simulink model "simulacao_modelos_discretos"  (R2018b)
settings: Solver=VariableStepAuto  StartTime=0.0  StopTime=15000  FixedStep=5  RelTol=1e-3
values from neighbouring files (symbols this model uses):
  sp_h3 = 0.48    [modelos.mat]    (also in termos_de_Ad.m = sp_h3*1e-2; validacao_tanques.m)
  sp_u = 33.8926009305    [modelos.mat]    (also in termos_de_Ad.m = (sp_q-357.3)/16.4; validacao_tanques.m = (sp_q-357.3)/16.4)
  T = 5.2632    [termos_de_Ad.m]
undefined symbols (not defined in the file or in its folder): Ad, Bd, Cd, Dd
settings Model: Creator=tarsis  LastModifiedBy=tarsis

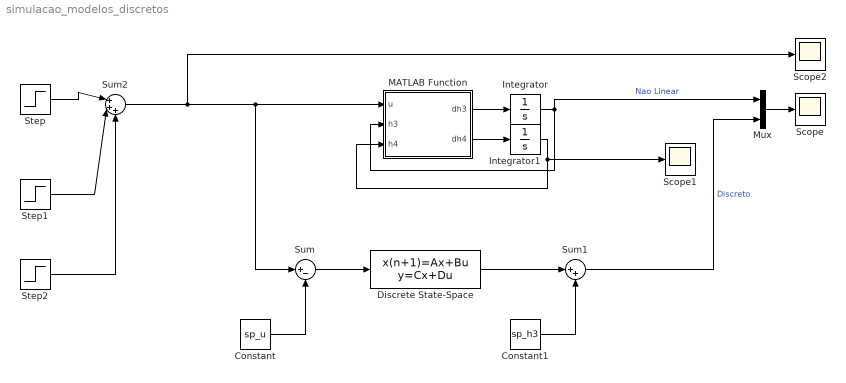
== system simulacao_modelos_discretos ==
  Constant : Constant  Value=sp_u
  Constant1 : Constant  Value=sp_h3
  Discrete State-Space : DiscreteStateSpace  A=Ad  B=Bd  C=Cd  D=Dd  SampleTime=T
  Integrator : Integrator
  Integrator1 : Integrator
  MATLAB Function : MATLAB Function  TreatAsAtomicUnit=on
  Mux : Mux  Inputs=2
  Scope : Scope
  Scope1 : Scope
  Scope2 : Scope
  Step : Step  Time=0  After=sp_u  SampleTime=T
  Step1 : Step  Time=5000  After=-sp_u*0.01  SampleTime=T
  Step2 : Step  Time=10000  After=sp_u*0.02  SampleTime=T
  Sum : Sum  Inputs=|+-
  Sum1 : Sum  Inputs=|++
  Sum2 : Sum  Inputs=|+++
  wires:
  MATLAB Function/1(dh3) -> Integrator/1
  MATLAB Function/2(dh4) -> Integrator1/1
  Integrator/1 -> Mux/1, MATLAB Function/2(h3)  "Nao Linear"
  Integrator1/1 -> Scope1/1, MATLAB Function/3(h4)
  Sum/1 -> Discrete State-Space/1
  Discrete State-Space/1 -> Sum1/1
  Constant/1 -> Sum/2
  Constant1/1 -> Sum1/2
  Mux/1 -> Scope/1
  Sum1/1 -> Mux/2  "Discreto"
  Step/1 -> Sum2/1
  Sum2/1 -> Scope2/1, Sum/1, MATLAB Function/1(u)
  Step1/1 -> Sum2/2
  Step2/1 -> Sum2/3

== matlab function simulacao_modelos_discretos/MATLAB Function ==
  data: u input; dh3 output; dh4 output; h3 input; h4 input
function [dh3,dh4] = fcn(u,h3,h4)
qi = (16.4*u + 357.3)*1e-6;
q12 = 33.51e-4*(h4 - h3) + 43.12e-5;
qout = (87.07e-5*sqrt(h3) + 30.99e-5);
A1 = (pi*(31)^2)*1e-4;
A2 = - 0.88629272879272778105782609278436*h3^16 + 6.0267905557905489111932174309337*h3^15 - 20.80464391736738395516887057851*h3^14 + 47.68494439008527766774004035511*h3^13 - 82.573907447205791291786792565001*h3^12 + 116.28257881925208875326233578017*h3^11 - 139.30893428077013388311346843447*h3^10 + 144.80767028205944702410747888441*h3^9 - 129.2475129476872169884635810807*h3^8 + 96.099152680911332924853135955618*h3^7 - 55.593870964701796673125553833866*h3^6 + 21.451550218200266654046211819752*h3^5 - 5.9275208717979510465216954484015*h3^4 + 3.9856416105248966168880953176109*h3^3 - 2.0902185091906828919771687989635*h3^2 - 0.061481774188906647716430580264178*h3 + 0.32722421068834535751546101783638;
dh4 = (qi - q12)/A1;
dh3 = (q12 - qout)/A2;
